simulink model "full_link"  (R2014b)
settings: Solver=ode45  StartTime=0.0  StopTime=20e-9  RelTol=1e-3
undefined symbols (not defined in the file or in its folder): UI
libraries: DesignElements x1, simulink x1
settings Model: Creator=Jase  LastModifiedBy=Jase

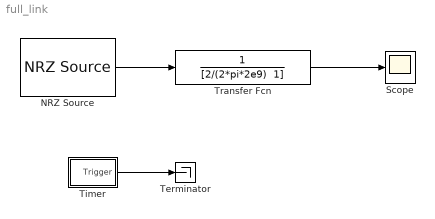
== system full_link ==
  NRZ Source : DesignElements/NRZ Source  Ts=UI
  Scope : Scope
  Terminator : Terminator
  Timer : Subsystem  mask{Time=1e-9}
      mask prompts: Time "Timer value"
  Transfer Fcn : TransferFcn  Denominator="[2/(2*pi*2e9)  1]"
  wires:
  NRZ Source/1 -> Transfer Fcn/1
  Transfer Fcn/1 -> Scope/1
  Timer/1(Trigger) -> Terminator/1

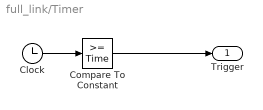
== system full_link/Timer ==
  Clock : Clock
  Compare To Constant : simulink/Logic and Bit Operations/Compare To Constant  relop=>=  const=Time  OutDataTypeStr=boolean
  Trigger : Outport
  wires:
  Compare To Constant/1 -> Trigger/1
  Clock/1 -> Compare To Constant/1
